simulink model "partE2"  (R2018b)
settings: Solver=VariableStepAuto  StartTime=0.0  StopTime=50  RelTol=1e-3
settings Model: Creator=amir  LastModifiedBy=amir

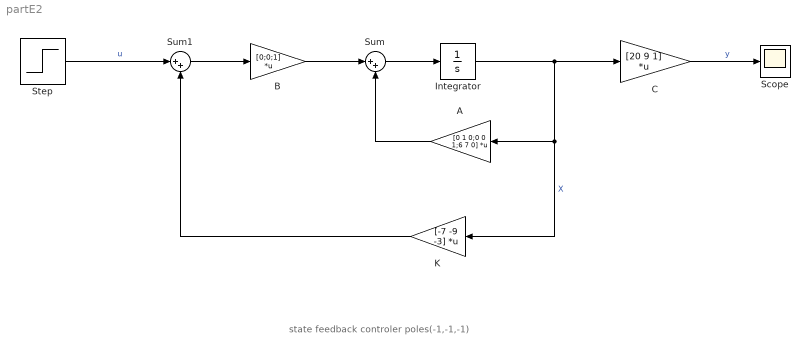
== system partE2 ==
  note: state feedback controler
      | poles(-1,-1,-1)
  A : Gain  Gain=[0 1 0;0 0 1;6 7 0]  Multiplication=Matrix(K*u) (u vector)
  B : Gain  Gain=[0;0;1]  Multiplication=Matrix(K*u) (u vector)
  C : Gain  Gain=[20 9 1]  Multiplication=Matrix(K*u) (u vector)
  Integrator : Integrator  InitialCondition=[1;1;1]
  K : Gain  Gain=[-7 -9 -3]  Multiplication=Matrix(K*u) (u vector)
  Scope : Scope
  Step : Step  After=20  SampleTime=0
  Sum : Sum  Inputs=|++
  Sum1 : Sum  Inputs=|++
  wires:
  B/1 -> Sum/1
  C/1 -> Scope/1  "y"
  Integrator/1 -> K/1, A/1, C/1  "X"
  A/1 -> Sum/2
  Sum/1 -> Integrator/1
  Sum1/1 -> B/1
  K/1 -> Sum1/2
  Step/1 -> Sum1/1  "u"
